simulink model "Satellite_Attitude_Model"  (R2018b)
settings: Solver=ode23tb  StartTime=0.0  StopTime=1000  FixedStep=0.001  RelTol=1e-4
values from neighbouring files (symbols this model uses):
  A = [A11, A12; A21, A22]    [Satellite_Attitude_Model_Parameters.m]
  ArgOfPerigee_init = deg2rad (TLE_degree(5))    [Satellite_Attitude_Model_Parameters.m]
  b = 10e-6    (= 1e-05)    [Satellite_Attitude_Model_Parameters.m]
  B = [B11,B12; B21,B22]    [Satellite_Attitude_Model_Parameters.m]
  D = 0    [Satellite_Attitude_Model_Parameters.m]
  eccentricity_init = TLE_degree(4)    [Satellite_Attitude_Model_Parameters.m]
  Hconf4 = [Hgyro;Hstr]    [Satellite_Attitude_Model_Parameters.m]
  inclination_init = deg2rad (TLE_degree(2))    [Satellite_Attitude_Model_Parameters.m]
  Km = 0.1    [Satellite_Attitude_Model_Parameters.m]
  Kt = 0.1    [Satellite_Attitude_Model_Parameters.m]
  L = 5.2e-3    (= 0.0052)    [Satellite_Attitude_Model_Parameters.m]
  MeanAnomaly_init = deg2rad (TLE_degree(6))    [Satellite_Attitude_Model_Parameters.m]
  meanMotion_init = meanMotion_init*2*pi/86400    [Satellite_Attitude_Model_Parameters.m]
  Q = 1e-10    [Satellite_Attitude_Model_Parameters.m]
  q_init = [0; 0; 0; 1]    [Satellite_Attitude_Model_Parameters.m]
  R = 2    [Satellite_Attitude_Model_Parameters.m]    (also in dynamicFunctions2.m = 7078000)
  RAAN_init = deg2rad (TLE_degree(3))    [Satellite_Attitude_Model_Parameters.m]
  Rconf4 = [diag(ones(3,1))*Rgyro zeros(3,4);         zeros(4,3) diag(ones(1,4))*Rstr]    [Satellite_Attitude_Model_Parameters.m]
  Rgyro = 1e-12    [Satellite_Attitude_Model_Parameters.m]
  Rstr = 1e-12    [Satellite_Attitude_Model_Parameters.m]
  rw_Inertia = 5e-4    (= 0.0005)    [Satellite_Attitude_Model_Parameters.m]
  RW_Mmax = 0.015    [Satellite_Attitude_Model_Parameters.m]
  rw_SensorToBody = [0 0.4741 0.4741 -0.9482;                   -0.9999 0.3333 0.3333 0.3333;                    0 -0.8165 0.8165 0 ]    [Satellite_Attitude_Model_Parameters.m]
  RW_wmax = 300    [Satellite_Attitude_Model_Parameters.m]
  satInertia = [Isx 0 0 ; 0 Isy 0 ; 0 0 Isz]    [Satellite_Attitude_Model_Parameters.m]    (also in dynamicFunctions2.m = diag([Isx Isy Isz]))
  semimajor_init = sqrt(mu_earth^(1/3)/meanMotion_init^(2/3))    [Satellite_Attitude_Model_Parameters.m]
  Ts = 0.01    [Satellite_Attitude_Model_Parameters.m]
  unit7 = ones(7,1)    [Satellite_Attitude_Model_Parameters.m]
  w_dot_init = [0;0;0]    [Satellite_Attitude_Model_Parameters.m]
  w_init = [0; 0; 0]    [Satellite_Attitude_Model_Parameters.m]
  wRW_init = [0;0;0;0]    [Satellite_Attitude_Model_Parameters.m]
undefined symbols (not defined in the file or in its folder): Continuous, Earth, Time, WGS84
libraries: simulink x14, simulink_extras x13, sharedtransform x8, aerolibutil x2, sharedTrackingLibrary x1, ctrlSharedLib x1, aerolibtransform2 x1, aerolibgravity2 x1
(part 2 of 3)

== system Satellite_Attitude_Model/Actuator Model (RW)/RW1 - DC Motor Controller3 ==
  RW1_Hdot_des : Inport
  Gain1 : Gain  Gain=12
  Gain2 : Gain  Gain=1/rw_Inertia
  Integrator : Integrator
  Mux : Mux  Inputs=2
  RW - DC Motor Model : Subsystem
  "Scope Desired and controlled RW-angular speed " : Scope
  Speed Controller1 : simulink/Continuous/PID Controller  Controller=PID  Form=Parallel  TimeDomain=Continuous-time  SampleTime=0.01  IntegratorMethod=Forward Euler  FilterMethod=Forward Euler  ControllerParametersSource=internal  P=9.56052273582853  I=13.4366327144231  D=1.16248121318414  UseFilter=on  N=2668.95305381072  TunerSelectOption=Transfer Function Based (PID Tuner App)  InitialConditionSource=internal  InitialConditionForIntegrator=0  InitialConditionForFilter=0  DifferentiatorICPrevScaledInput=0  ExternalReset=none  TrackingMode=off  Kt=1  LimitOutput=off  UpperSaturationLimit=inf  LowerSaturationLimit=-inf  LinearizeAsGain=on  AntiWindupMode=none  Kb=1  POutMin=[]  POutMax=[]  IOutMin=[]  IOutMax=[]  DOutMin=[]  DOutMax=[]  NOutMin=[]  NOutMax=[]  SumOutMin=[]  SumOutMax=[]  SaturationOutMin=[]  SaturationOutMax=[]  PParamMin=[]  PParamMax=[]  IParamMin=[]  IParamMax=[]  DParamMin=[]  DParamMax=[]  NParamMin=[]  NParamMax=[]  KbParamMin=[]  KbParamMax=[]  KtParamMin=[]  KtParamMax=[]  KbOutMin=[]  KbOutMax=[]  KtOutMin=[]  KtOutMax=[]  IntegratorOutMin=[]  IntegratorOutMax=[]  FilterOutMin=[]  FilterOutMax=[]  SumI1OutMin=[]  SumI1OutMax=[]  SumI2OutMin=[]  SumI2OutMax=[]  SumI3OutMin=[]  SumI3OutMax=[]  SumI4OutMin=[]  SumI4OutMax=[]  SumDOutMin=[]  SumDOutMax=[]  DifferentiatorOutMin=[]  DifferentiatorOutMax=[]  FilterDiffOutCoefMin=[]  FilterDiffOutCoefMax=[]  ReciprocalOutMin=[]  ReciprocalOutMax=[]  SumDenOutMin=[]  SumDenOutMax=[]  SumNumOutMin=[]  SumNumOutMax=[]  DivideOutMin=[]  DivideOutMax=[]  IntegratorContinuousStateAttributes=''  IntegratorStateMustResolveToSignalObject=off  IntegratorRTWStateStorageClass=Auto  FilterContinuousStateAttributes=''  FilterStateMustResolveToSignalObject=off  FilterRTWStateStorageClass=Auto  ParallelPVariant=InternalParameters  IdealPVariant=Disabled  IVariant=InternalParameters  DVariant=InternalParameters  IntegratorVariant=Continuous  SatVariant=Disabled  AWVariant=Passthrough  PCopyVariant=Disabled  TRVariant=Disabled  FdbkBlocksVariant=Forward  IdealPFdbkVariant=Disabled  SatFdbkVariant=Disabled  DerivativeFilterVariant=ContFilter  NVariant=InternalParameters  NCopyVariant=Disabled  FilterICVariant=InternalICsFilter  IntegratorICVariant=InternalICs  ExternalResetVariant=Disabled  TRSumVariant=Passthrough  SumFdbkVariant=Disabled  SumVariant=Sum_PID
  Sum1 : Sum  Inputs=|+-
  Sum2 : Sum  Inputs=|+-
  Torque Controller : simulink/Continuous/PID Controller  Controller=PID  Form=Parallel  TimeDomain=Continuous-time  SampleTime=0.01  IntegratorMethod=Forward Euler  FilterMethod=Forward Euler  ControllerParametersSource=internal  P=2.50374683332827e-05  I=0.022215359014968  D=0  UseFilter=on  N=100  TunerSelectOption=Transfer Function Based (PID Tuner App)  InitialConditionSource=internal  InitialConditionForIntegrator=0  InitialConditionForFilter=0  DifferentiatorICPrevScaledInput=0  ExternalReset=none  TrackingMode=off  Kt=1  LimitOutput=off  UpperSaturationLimit=inf  LowerSaturationLimit=-inf  LinearizeAsGain=on  AntiWindupMode=none  Kb=1  POutMin=[]  POutMax=[]  IOutMin=[]  IOutMax=[]  DOutMin=[]  DOutMax=[]  NOutMin=[]  NOutMax=[]  SumOutMin=[]  SumOutMax=[]  SaturationOutMin=[]  SaturationOutMax=[]  PParamMin=[]  PParamMax=[]  IParamMin=[]  IParamMax=[]  DParamMin=[]  DParamMax=[]  NParamMin=[]  NParamMax=[]  KbParamMin=[]  KbParamMax=[]  KtParamMin=[]  KtParamMax=[]  KbOutMin=[]  KbOutMax=[]  KtOutMin=[]  KtOutMax=[]  IntegratorOutMin=[]  IntegratorOutMax=[]  FilterOutMin=[]  FilterOutMax=[]  SumI1OutMin=[]  SumI1OutMax=[]  SumI2OutMin=[]  SumI2OutMax=[]  SumI3OutMin=[]  SumI3OutMax=[]  SumI4OutMin=[]  SumI4OutMax=[]  SumDOutMin=[]  SumDOutMax=[]  DifferentiatorOutMin=[]  DifferentiatorOutMax=[]  FilterDiffOutCoefMin=[]  FilterDiffOutCoefMax=[]  ReciprocalOutMin=[]  ReciprocalOutMax=[]  SumDenOutMin=[]  SumDenOutMax=[]  SumNumOutMin=[]  SumNumOutMax=[]  DivideOutMin=[]  DivideOutMax=[]  IntegratorContinuousStateAttributes=''  IntegratorStateMustResolveToSignalObject=off  IntegratorRTWStateStorageClass=Auto  FilterContinuousStateAttributes=''  FilterStateMustResolveToSignalObject=off  FilterRTWStateStorageClass=Auto  ParallelPVariant=InternalParameters  IdealPVariant=Disabled  IVariant=InternalParameters  DVariant=InternalParameters  IntegratorVariant=Continuous  SatVariant=Disabled  AWVariant=Passthrough  PCopyVariant=Disabled  TRVariant=Disabled  FdbkBlocksVariant=Forward  IdealPFdbkVariant=Disabled  SatFdbkVariant=Disabled  DerivativeFilterVariant=ContFilter  NVariant=InternalParameters  NCopyVariant=Disabled  FilterICVariant=InternalICsFilter  IntegratorICVariant=InternalICs  ExternalResetVariant=Disabled  TRSumVariant=Passthrough  SumFdbkVariant=Disabled  SumVariant=Sum_PID
  V limit : Saturate  UpperLimit=20  LowerLimit=-20
  w limit : Saturate  UpperLimit=RW_wmax  LowerLimit=-RW_wmax
  RW1_H : Outport
  RW1_w : Outport  Port=2
  RW1_Hdot : Outport  Port=3
  wires:
  Torque Controller/1 -> V limit/1
  RW - DC Motor Model/3(RW_Hrw_dot) -> RW1_Hdot/1, Sum1/2
  Mux/1 -> "Scope Desired and controlled RW-angular speed "/1
  V limit/1 -> Gain1/1
  Gain1/1 -> RW - DC Motor Model/1(V-rw)  "V-rw"
  RW - DC Motor Model/2(RW_w) -> RW1_w/1, Sum2/2, Mux/2
  Sum1/1 -> Torque Controller/1
  RW - DC Motor Model/1(RW_Hrw) -> RW1_H/1
  Speed Controller1/1 -> w limit/1
  w limit/1 -> Sum1/1
  Sum2/1 -> Speed Controller1/1  "M-error"
  Integrator/1 -> Gain2/1
  RW1_Hdot_des/1 -> Integrator/1
  Gain2/1 -> Mux/1, Sum2/1

== system Satellite_Attitude_Model/Actuator Model (RW)/RW1 - DC Motor Controller5 ==
  RW1_Hdot_des : Inport
  Gain1 : Gain  Gain=12
  Gain2 : Gain  Gain=1/rw_Inertia
  Integrator : Integrator
  Mux : Mux  Inputs=2
  RW - DC Motor Model : Subsystem
  "Scope Desired and controlled RW-angular speed " : Scope
  Speed Controller1 : simulink/Continuous/PID Controller  Controller=PID  Form=Parallel  TimeDomain=Continuous-time  SampleTime=0.01  IntegratorMethod=Forward Euler  FilterMethod=Forward Euler  ControllerParametersSource=internal  P=9.56052273582853  I=13.4366327144231  D=1.16248121318414  UseFilter=on  N=2668.95305381072  TunerSelectOption=Transfer Function Based (PID Tuner App)  InitialConditionSource=internal  InitialConditionForIntegrator=0  InitialConditionForFilter=0  DifferentiatorICPrevScaledInput=0  ExternalReset=none  TrackingMode=off  Kt=1  LimitOutput=off  UpperSaturationLimit=inf  LowerSaturationLimit=-inf  LinearizeAsGain=on  AntiWindupMode=none  Kb=1  POutMin=[]  POutMax=[]  IOutMin=[]  IOutMax=[]  DOutMin=[]  DOutMax=[]  NOutMin=[]  NOutMax=[]  SumOutMin=[]  SumOutMax=[]  SaturationOutMin=[]  SaturationOutMax=[]  PParamMin=[]  PParamMax=[]  IParamMin=[]  IParamMax=[]  DParamMin=[]  DParamMax=[]  NParamMin=[]  NParamMax=[]  KbParamMin=[]  KbParamMax=[]  KtParamMin=[]  KtParamMax=[]  KbOutMin=[]  KbOutMax=[]  KtOutMin=[]  KtOutMax=[]  IntegratorOutMin=[]  IntegratorOutMax=[]  FilterOutMin=[]  FilterOutMax=[]  SumI1OutMin=[]  SumI1OutMax=[]  SumI2OutMin=[]  SumI2OutMax=[]  SumI3OutMin=[]  SumI3OutMax=[]  SumI4OutMin=[]  SumI4OutMax=[]  SumDOutMin=[]  SumDOutMax=[]  DifferentiatorOutMin=[]  DifferentiatorOutMax=[]  FilterDiffOutCoefMin=[]  FilterDiffOutCoefMax=[]  ReciprocalOutMin=[]  ReciprocalOutMax=[]  SumDenOutMin=[]  SumDenOutMax=[]  SumNumOutMin=[]  SumNumOutMax=[]  DivideOutMin=[]  DivideOutMax=[]  IntegratorContinuousStateAttributes=''  IntegratorStateMustResolveToSignalObject=off  IntegratorRTWStateStorageClass=Auto  FilterContinuousStateAttributes=''  FilterStateMustResolveToSignalObject=off  FilterRTWStateStorageClass=Auto  ParallelPVariant=InternalParameters  IdealPVariant=Disabled  IVariant=InternalParameters  DVariant=InternalParameters  IntegratorVariant=Continuous  SatVariant=Disabled  AWVariant=Passthrough  PCopyVariant=Disabled  TRVariant=Disabled  FdbkBlocksVariant=Forward  IdealPFdbkVariant=Disabled  SatFdbkVariant=Disabled  DerivativeFilterVariant=ContFilter  NVariant=InternalParameters  NCopyVariant=Disabled  FilterICVariant=InternalICsFilter  IntegratorICVariant=InternalICs  ExternalResetVariant=Disabled  TRSumVariant=Passthrough  SumFdbkVariant=Disabled  SumVariant=Sum_PID
  Sum1 : Sum  Inputs=|+-
  Sum2 : Sum  Inputs=|+-
  Torque Controller : simulink/Continuous/PID Controller  Controller=PID  Form=Parallel  TimeDomain=Continuous-time  SampleTime=0.01  IntegratorMethod=Forward Euler  FilterMethod=Forward Euler  ControllerParametersSource=internal  P=2.50374683332827e-05  I=0.022215359014968  D=0  UseFilter=on  N=100  TunerSelectOption=Transfer Function Based (PID Tuner App)  InitialConditionSource=internal  InitialConditionForIntegrator=0  InitialConditionForFilter=0  DifferentiatorICPrevScaledInput=0  ExternalReset=none  TrackingMode=off  Kt=1  LimitOutput=off  UpperSaturationLimit=inf  LowerSaturationLimit=-inf  LinearizeAsGain=on  AntiWindupMode=none  Kb=1  POutMin=[]  POutMax=[]  IOutMin=[]  IOutMax=[]  DOutMin=[]  DOutMax=[]  NOutMin=[]  NOutMax=[]  SumOutMin=[]  SumOutMax=[]  SaturationOutMin=[]  SaturationOutMax=[]  PParamMin=[]  PParamMax=[]  IParamMin=[]  IParamMax=[]  DParamMin=[]  DParamMax=[]  NParamMin=[]  NParamMax=[]  KbParamMin=[]  KbParamMax=[]  KtParamMin=[]  KtParamMax=[]  KbOutMin=[]  KbOutMax=[]  KtOutMin=[]  KtOutMax=[]  IntegratorOutMin=[]  IntegratorOutMax=[]  FilterOutMin=[]  FilterOutMax=[]  SumI1OutMin=[]  SumI1OutMax=[]  SumI2OutMin=[]  SumI2OutMax=[]  SumI3OutMin=[]  SumI3OutMax=[]  SumI4OutMin=[]  SumI4OutMax=[]  SumDOutMin=[]  SumDOutMax=[]  DifferentiatorOutMin=[]  DifferentiatorOutMax=[]  FilterDiffOutCoefMin=[]  FilterDiffOutCoefMax=[]  ReciprocalOutMin=[]  ReciprocalOutMax=[]  SumDenOutMin=[]  SumDenOutMax=[]  SumNumOutMin=[]  SumNumOutMax=[]  DivideOutMin=[]  DivideOutMax=[]  IntegratorContinuousStateAttributes=''  IntegratorStateMustResolveToSignalObject=off  IntegratorRTWStateStorageClass=Auto  FilterContinuousStateAttributes=''  FilterStateMustResolveToSignalObject=off  FilterRTWStateStorageClass=Auto  ParallelPVariant=InternalParameters  IdealPVariant=Disabled  IVariant=InternalParameters  DVariant=InternalParameters  IntegratorVariant=Continuous  SatVariant=Disabled  AWVariant=Passthrough  PCopyVariant=Disabled  TRVariant=Disabled  FdbkBlocksVariant=Forward  IdealPFdbkVariant=Disabled  SatFdbkVariant=Disabled  DerivativeFilterVariant=ContFilter  NVariant=InternalParameters  NCopyVariant=Disabled  FilterICVariant=InternalICsFilter  IntegratorICVariant=InternalICs  ExternalResetVariant=Disabled  TRSumVariant=Passthrough  SumFdbkVariant=Disabled  SumVariant=Sum_PID
  V limit : Saturate  UpperLimit=20  LowerLimit=-20
  w limit : Saturate  UpperLimit=RW_wmax  LowerLimit=-RW_wmax
  RW1_H : Outport
  RW1_w : Outport  Port=2
  RW1_Hdot : Outport  Port=3
  wires:
  Torque Controller/1 -> V limit/1
  RW - DC Motor Model/3(RW_Hrw_dot) -> RW1_Hdot/1, Sum1/2
  Mux/1 -> "Scope Desired and controlled RW-angular speed "/1
  V limit/1 -> Gain1/1
  Gain1/1 -> RW - DC Motor Model/1(V-rw)  "V-rw"
  RW - DC Motor Model/2(RW_w) -> RW1_w/1, Sum2/2, Mux/2
  Sum1/1 -> Torque Controller/1
  RW - DC Motor Model/1(RW_Hrw) -> RW1_H/1
  Speed Controller1/1 -> w limit/1
  w limit/1 -> Sum1/1
  Sum2/1 -> Speed Controller1/1  "M-error"
  Integrator/1 -> Gain2/1
  RW1_Hdot_des/1 -> Integrator/1
  Gain2/1 -> Mux/1, Sum2/1

== system Satellite_Attitude_Model/Julian Date Model/Time To Julian Date Model ==
  time : Inport
  Date To Julian Date Model : MATLAB Function  TreatAsAtomicUnit=on
  JulianDate : Outport
  wires:
  time/1 -> Date To Julian Date Model/1(time)
  Date To Julian Date Model/1(JD) -> JulianDate/1

== system Satellite_Attitude_Model/Orbit Propagator Model/Mean Motion To Semi-major Axis ==
  In1 : Inport
  MATLAB Function : MATLAB Function  TreatAsAtomicUnit=on
  Out1 : Outport
  wires:
  In1/1 -> MATLAB Function/1(a)
  MATLAB Function/1(meanMotion) -> Out1/1

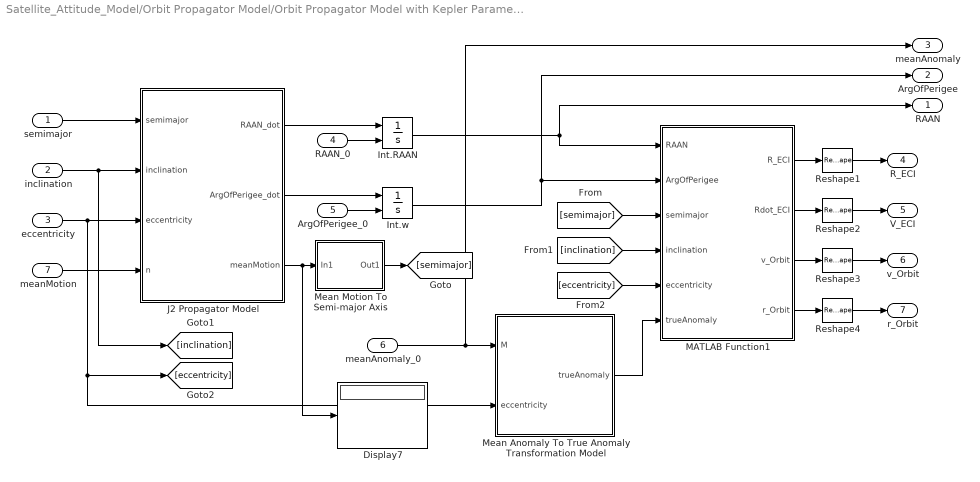
== system Satellite_Attitude_Model/Orbit Propagator Model/Orbit Propagator Model with Kepler Parameters(ECI) ==
  semimajor : Inport
  inclination : Inport  Port=2
  eccentricity : Inport  Port=3
  RAAN_0 : Inport  Port=4
  ArgOfPerigee_0 : Inport  Port=5
  meanAnomaly_0 : Inport  Port=6
  meanMotion : Inport  Port=7
  Display7 : Display
  Int.RAAN : Integrator  InitialConditionSource=external
  Int.w : Integrator  InitialConditionSource=external
  J2 Propagator Model : MATLAB Function  TreatAsAtomicUnit=on
  MATLAB Function1 : MATLAB Function  TreatAsAtomicUnit=on
  Mean Anomaly To True Anomaly Transformation Model : MATLAB Function  TreatAsAtomicUnit=on
  Mean Motion To Semi-major Axis : Subsystem
  Reshape{1..4} (4 alike) : Reshape  OutputDimensionality=Column vector (2-D)
  RAAN : Outport
  ArgOfPerigee : Outport  Port=2
  meanAnomaly : Outport  Port=3
  R_ECI : Outport  Port=4
  V_ECI : Outport  Port=5
  v_Orbit : Outport  Port=6
  r_Orbit : Outport  Port=7
  wires:
  ArgOfPerigee_0/1 -> Int.w/2
  RAAN_0/1 -> Int.RAAN/2
  semimajor/1 -> J2 Propagator Model/1(semimajor)
  J2 Propagator Model/2(ArgOfPerigee_dot) -> Int.w/1
  J2 Propagator Model/1(RAAN_dot) -> Int.RAAN/1
  Int.RAAN/1 -> MATLAB Function1/1(RAAN), RAAN/1
  Int.w/1 -> ArgOfPerigee/1, MATLAB Function1/2(ArgOfPerigee)
  meanAnomaly_0/1 -> meanAnomaly/1, Mean Anomaly To True Anomaly Transformation Model/1(M)
  inclination/1 -> [inclination], J2 Propagator Model/2(inclination)
  eccentricity/1 -> Mean Anomaly To True Anomaly Transformation Model/2(eccentricity), [eccentricity], J2 Propagator Model/3(eccentricity)
  Mean Anomaly To True Anomaly Transformation Model/1(trueAnomaly) -> MATLAB Function1/6(trueAnomaly)
  MATLAB Function1/2(Rdot_ECI) -> Reshape2/1
  MATLAB Function1/1(R_ECI) -> Reshape1/1
  Reshape2/1 -> V_ECI/1
  Reshape1/1 -> R_ECI/1
  [semimajor] -> MATLAB Function1/3(semimajor)
  [inclination] -> MATLAB Function1/4(inclination)
  [eccentricity] -> MATLAB Function1/5(eccentricity)
  MATLAB Function1/3(v_Orbit) -> Reshape3/1
  Reshape3/1 -> v_Orbit/1
  MATLAB Function1/4(r_Orbit) -> Reshape4/1
  Reshape4/1 -> r_Orbit/1
  meanMotion/1 -> J2 Propagator Model/4(n)
  Mean Motion To Semi-major Axis/1(Out1) -> [semimajor]
  J2 Propagator Model/3(meanMotion) -> Display7/1, Mean Motion To Semi-major Axis/1(In1)

== system Satellite_Attitude_Model/Orbit Propagator Model/True Anomaly to Mean Anomaly ==
  ecc : Inport
  TrAn : Inport  Port=2
  True Anomaly to Mean Anomaly : MATLAB Function  TreatAsAtomicUnit=on
  Out1 : Outport
  wires:
  TrAn/1 -> True Anomaly to Mean Anomaly/2(TrAn)
  ecc/1 -> True Anomaly to Mean Anomaly/1(ecc)
  True Anomaly to Mean Anomaly/1(M) -> Out1/1

== system Satellite_Attitude_Model/Satellite Kinematic & Dynamic Model/Dynamic Model ==
  Mc+Md : Inport
  "Hrw_B " : Inport  Port=2
  Add : Sum  Inputs=-+
  Add1 : Sum
  Embedded MATLAB Function : MATLAB Function  TreatAsAtomicUnit=on
  IC : InitialCondition  Value=w_init
  IC1 : InitialCondition  Value=w_dot_init
  Inertia Matrix : Constant  Value=satInertia  VectorParams1D=off
  Integrator : Integrator  InitialConditionSource=external  InitialCondition=[0;0;0]
  Invert 3x3 Matrix : aerolibutil/Invert  3x3 Matrix
  Product : Product  Multiplication=Matrix(*)  RndMeth=Zero
  Product1 : Product  Multiplication=Matrix(*)  RndMeth=Zero
  Reshape : Reshape  OutputDimensionality=Column vector (2-D)
  Reshape1 : Reshape  OutputDimensionality=Column vector (2-D)
  w_initial : Constant  Value=w_init  VectorParams1D=off  SampleTime=-1
  w_IB_B : Outport
  wires:
  Inertia Matrix/1 -> Invert 3x3 Matrix/1, Product/1
  IC/1 -> Product/2, Embedded MATLAB Function/1(w)
  Mc+Md/1 -> Reshape1/1
  Invert 3x3 Matrix/1 -> Product1/1
  Integrator/1 -> w_IB_B/1, IC/1
  Product1/1 -> IC1/1
  Embedded MATLAB Function/1(y) -> Reshape/1
  w_initial/1 -> Integrator/2
  Add/1 -> Product1/2
  IC1/1 -> Integrator/1
  Reshape/1 -> Add/1
  Reshape1/1 -> Add/2
  Product/1 -> Add1/1
  Add1/1 -> Embedded MATLAB Function/2(Iw_plus_hwheel)
  "Hrw_B "/1 -> Add1/2

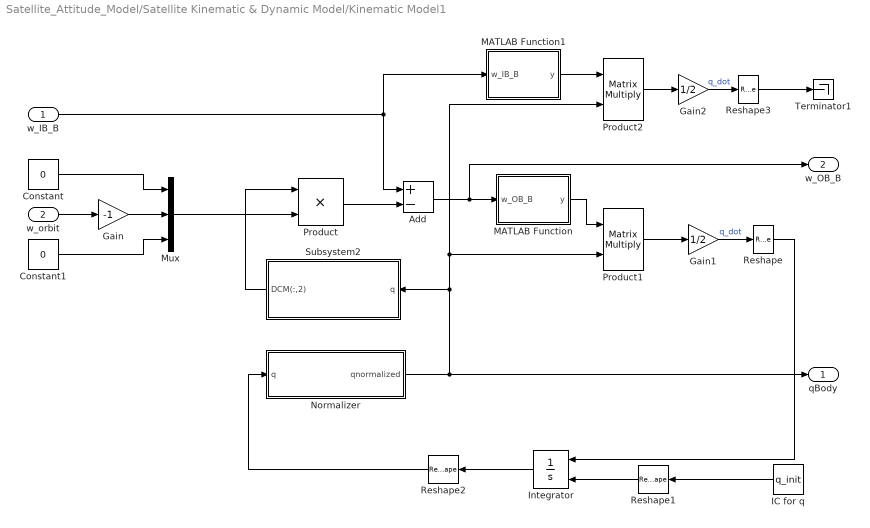
== system Satellite_Attitude_Model/Satellite Kinematic & Dynamic Model/Kinematic Model1 ==
  w_IB_B : Inport
  w_orbit : Inport  Port=2
  Add : Sum  Inputs=+-
  Constant : Constant  Value=0
  Constant1 : Constant  Value=0
  Gain : Gain  Gain=-1
  Gain1 : Gain  Gain=1/2
  Gain2 : Gain  Gain=1/2
  IC for q : Constant  Value=q_init  SampleTime=Ts
  Integrator : Integrator  InitialConditionSource=external
  MATLAB Function : MATLAB Function  TreatAsAtomicUnit=on
  MATLAB Function1 : MATLAB Function  TreatAsAtomicUnit=on
  Mux : Mux  Inputs=3
  Normalizer : MATLAB Function  TreatAsAtomicUnit=on
  Product : Product
  Product1 : Product  Multiplication=Matrix(*)
  Product2 : Product  Multiplication=Matrix(*)
  Reshape{,1..3} (4 alike) : Reshape  OutputDimensionality=Column vector (2-D)
  Subsystem2 : Subsystem
  Terminator1 : Terminator
  qBody : Outport
  w_OB_B : Outport  Port=2
  wires:
  Reshape2/1 -> Normalizer/1(q)
  Product/1 -> Add/2
  Integrator/1 -> Reshape2/1
  Normalizer/1(qnormalized) -> qBody/1, Subsystem2/1(q), Product1/2, Product2/2
  IC for q/1 -> Reshape1/1
  Reshape1/1 -> Integrator/2
  Add/1 -> MATLAB Function/1(w_OB_B), w_OB_B/1
  w_orbit/1 -> Gain/1
  Mux/1 -> Product/2
  Constant/1 -> Mux/1
  Constant1/1 -> Mux/3
  Product1/1 -> Gain1/1
  MATLAB Function/1(y) -> Product1/1
  Gain1/1 -> Reshape/1  "q_dot"
  w_IB_B/1 -> MATLAB Function1/1(w_IB_B), Add/1
  Product2/1 -> Gain2/1
  MATLAB Function1/1(y) -> Product2/1
  Gain2/1 -> Reshape3/1  "q_dot"
  Subsystem2/1(DCM(:,2)) -> Product/1
  Gain/1 -> Mux/2
  Reshape/1 -> Integrator/1
  Reshape3/1 -> Terminator1/1

== system Satellite_Attitude_Model/Satellite Kinematic & Dynamic Model/Subsystem ==
  qest : Inport
  Quaternions to Direction Cosine Matrix : sharedtransform/Quaternions to  Direction Cosine Matrix  aMode=aMode
      settings: SourceProductName=Aerospace Blockset  SourceProductBaseCode=AE
  Subsystem : Subsystem
  "DCM " : Outport
  wires:
  Quaternions to Direction Cosine Matrix/1 -> "DCM "/1
  Subsystem/1(q0,q1,q2,q3) -> Quaternions to Direction Cosine Matrix/1
  qest/1 -> Subsystem/1(q1,q2,q3,q4)

== system Satellite_Attitude_Model/Satellite Kinematic & Dynamic Model/Subsystem1 ==
  "DCM " : Inport
  Direction Cosine Matrix to Rotation Angles : sharedtransform/Direction Cosine Matrix to Rotation Angles  rotationOrder=ZYX  aMode=aMode  action=None  tolerance=eps(2)
      settings: SourceProductName=Aerospace Blockset  SourceProductBaseCode=AE
  Radians to Degrees1 : simulink_extras/Transformations/Radians to Degrees
  Euler Angle : Outport
  wires:
  Radians to Degrees1/1 -> Euler Angle/1
  Direction Cosine Matrix to Rotation Angles/1 -> Radians to Degrees1/1
  "DCM "/1 -> Direction Cosine Matrix to Rotation Angles/1

== system Satellite_Attitude_Model/Sensor Measurement Model (GYRO + STR)/GYRO Sensor Model ==
  w_Body : Inport
  Gyroscope Model : Subsystem
  Zero-Order Hold2 : ZeroOrderHold  SampleTime=Ts
  w_Body_meas : Outport
  wires:
  w_Body/1 -> Gyroscope Model/1(w_Body)
  Gyroscope Model/1(Gyro1_wmeas) -> Zero-Order Hold2/1
  Zero-Order Hold2/1 -> w_Body_meas/1

== system Satellite_Attitude_Model/Sensor Measurement Model (GYRO + STR)/Normalization Model ==
  u : Inport
  Divide : Product  Inputs=*/
  MATLAB Function : MATLAB Function  TreatAsAtomicUnit=on
  Math Function2 : Math  Operator=square  SaturateOnIntegerOverflow=on
  Sum of Elements : Sum  Inputs=+
  Normalized_u : Outport
  wires:
  Divide/1 -> Normalized_u/1
  MATLAB Function/1(y) -> Divide/2
  Sum of Elements/1 -> MATLAB Function/1(u)
  u/1 -> Divide/1, Math Function2/1
  Math Function2/1 -> Sum of Elements/1

== system Satellite_Attitude_Model/Sensor Measurement Model (GYRO + STR)/Star Tracker Model ==
  q_Body : Inport
  Scope : Scope
  StarTracker 1 Error Model3 : Subsystem  TreatAsAtomicUnit=on
  Zero-Order Hold2 : ZeroOrderHold  SampleTime=0.1
  q_Body_meas : Outport
  wires:
  Zero-Order Hold2/1 -> Scope/1, q_Body_meas/1
  q_Body/1 -> StarTracker 1 Error Model3/1("q_Body ")
  StarTracker 1 Error Model3/1("q_body_meas ") -> Zero-Order Hold2/1

== system Satellite_Attitude_Model/Subsystem/Subsystem1 ==
  q0,q1,q2,q3 : Inport
  Demux1 : Demux
  Mux1 : Mux
  q1,q2,q3,q4 : Outport
  wires:
  q0,q1,q2,q3/1 -> Demux1/1
  Mux1/1 -> q1,q2,q3,q4/1
  Demux1/1 -> Mux1/4
  Demux1/2 -> Mux1/1
  Demux1/3 -> Mux1/2
  Demux1/4 -> Mux1/3

== system Satellite_Attitude_Model/Subsystem2/Subsystem ==
  qest : Inport
  Demux2 : Demux
  Mux2 : Mux
  Quaternions to Direction Cosine Matrix : sharedtransform/Quaternions to  Direction Cosine Matrix  aMode=aMode
      settings: SourceProductName=Aerospace Blockset  SourceProductBaseCode=AE
  "DCM " : Outport
  wires:
  Mux2/1 -> Quaternions to Direction Cosine Matrix/1
  Quaternions to Direction Cosine Matrix/1 -> "DCM "/1
  Demux2/2 -> Mux2/3
  Demux2/4 -> Mux2/1
  Demux2/3 -> Mux2/4
  Demux2/1 -> Mux2/2
  qest/1 -> Demux2/1

== system Satellite_Attitude_Model/Sun Position Model/Subsystem1 ==
  JD2000 : Inport
  r_ECI : Inport  Port=2
  DCM_qECI : Inport  Port=3
  DCM_qBody : Inport  Port=4
  Display3 : Display
  Invert 3x3 Matrix : aerolibutil/Invert  3x3 Matrix
  Product : Product  Multiplication=Matrix(*)
  Product1 : Product  Multiplication=Matrix(*)
  "Sun Vector Model " : Subsystem
  SunVector_Orbit : Outport
  "sunVector_ECI " : Outport  Port=2
  wires:
  "Sun Vector Model "/1(sunVector_ECI) -> "sunVector_ECI "/1, Product/2, Display3/1
  JD2000/1 -> "Sun Vector Model "/1(JD2000)
  Product/1 -> Product1/2
  Product1/1 -> SunVector_Orbit/1
  Invert 3x3 Matrix/1 -> Product1/1
  DCM_qECI/1 -> Product/1
  DCM_qBody/1 -> Invert 3x3 Matrix/1
  r_ECI/1 -> "Sun Vector Model "/2(rECI)

== system Satellite_Attitude_Model/Total Disturbance Torque Model/Aerodynamic Disturbance Torque Model ==
  SC_Velocity_Orbit : Inport
  DCM : Inport  Port=2
  Aerodynamic Disturbance Torque Model : Subsystem
  Product : Product  Multiplication=Matrix(*)
  AerodynamicDistTorque_Orbit : Outport
  AerodynamicDistTorque_Body : Outport  Port=2
  wires:
  Aerodynamic Disturbance Torque Model/1(AerodynamicDistTorque) -> Product/2, AerodynamicDistTorque_Orbit/1
  Product/1 -> AerodynamicDistTorque_Body/1
  DCM/1 -> Product/1
  SC_Velocity_Orbit/1 -> Aerodynamic Disturbance Torque Model/1(SC_Velocity_Orbit)

== system Satellite_Attitude_Model/Total Disturbance Torque Model/Gravity Gradient Disturbance Torque Model ==
  w0 : Inport
  DCM : Inport  Port=2
  SatInertiaMatrix : Inport  Port=3
  Gain : Gain  Gain=3
  "Last Column " : MATLAB Function  TreatAsAtomicUnit=on
  Product : Product
  Product1 : Product
  Product2 : Product  Multiplication=Matrix(*)
  Product3 : Product  Multiplication=Matrix(*)
  Product4 : Product  Multiplication=Matrix(*)
  Skew Symmetric Matrix : MATLAB Function  TreatAsAtomicUnit=on
  GGDistTorque : Outport
  GGDistTorque_Body : Outport  Port=2
  wires:
  Gain/1 -> Product1/1
  Product2/1 -> Product3/2  "3x1"
  w0/1 -> Product/1, Product/2
  Product3/1 -> Product1/2
  Product1/1 -> Product4/2, GGDistTorque/1
  "Last Column "/1(LastColumn_DCM) -> Product2/2, Skew Symmetric Matrix/1(LastColumn_DCM)  "3x1"
  Product/1 -> Gain/1
  SatInertiaMatrix/1 -> Product2/1
  Skew Symmetric Matrix/1(SkewSym_DCM) -> Product3/1  "3x3"
  DCM/1 -> Product4/1, "Last Column "/1(DCM)
  Product4/1 -> GGDistTorque_Body/1

== system Satellite_Attitude_Model/Total Disturbance Torque Model/Magnetic Field Disturbance Torque Model ==
  LLA_degrees : Inport
  DCM_qBody : Inport  Port=2
  Subsystem : Subsystem
  MagFieldDistTorque_Orbit : Outport
  MagFieldDistTorque_Body : Outport  Port=2
  wires:
  Subsystem/1(MagField_Orbit) -> MagFieldDistTorque_Orbit/1
  Subsystem/2(MagField_Body) -> MagFieldDistTorque_Body/1
  LLA_degrees/1 -> Subsystem/1(LLA_degrees)
  DCM_qBody/1 -> Subsystem/2(DCM_qBody)

== system Satellite_Attitude_Model/Total Disturbance Torque Model/Solar Radiation Disturbance Torque Model ==
  SunVector_Orbit : Inport
  DCM : Inport  Port=2
  Product : Product  Multiplication=Matrix(*)
  Solar Radiation Disturbance Torque Model : Subsystem
  SolarRadDistTorque : Outport
  SolarRadDistTorque_Body : Outport  Port=2
  wires:
  SunVector_Orbit/1 -> Solar Radiation Disturbance Torque Model/1(SunPositionVector)
  Solar Radiation Disturbance Torque Model/1(SolarRadDistTorque) -> SolarRadDistTorque/1, Product/2
  Product/1 -> SolarRadDistTorque_Body/1
  DCM/1 -> Product/1

== system Satellite_Attitude_Model/Actuator Model (RW)/RW1 - DC Motor Controller1/RW - DC Motor Model ==
  V-rw : Inport
  Gain : Gain  Gain=Km
  Gain2 : Gain  Gain=Kt
  Gain6 : Gain  Gain=rw_Inertia
  M(s) --> w(s) : simulink_extras/Additional Linear/Transfer Fcn (with initial states)  N=[1]  D=[rw_Inertia b]  X0=0
  Sum3 : Sum  Inputs=|+-
  V(s) --> I(s) : simulink_extras/Additional Linear/Transfer Fcn (with initial states)  N=1  D=[L R]  X0=0
  w limit : Saturate  UpperLimit=RW_wmax  LowerLimit=-RW_wmax
  RW_Hrw : Outport
  RW_w : Outport  Port=2
  RW_Hrw_dot : Outport  Port=3
  wires:
  V-rw/1 -> Sum3/1
  Gain2/1 -> M(s) --> w(s)/1, RW_Hrw_dot/1  "M-rw"
  Gain6/1 -> RW_Hrw/1
  Gain/1 -> Sum3/2
  M(s) --> w(s)/1 -> w limit/1
  Sum3/1 -> V(s) --> I(s)/1  "V-rw"
  V(s) --> I(s)/1 -> Gain2/1
  w limit/1 -> RW_w/1, Gain6/1, Gain/1

== system Satellite_Attitude_Model/Actuator Model (RW)/RW1 - DC Motor Controller2/RW - DC Motor Model ==
  V-rw : Inport
  Gain : Gain  Gain=Km
  Gain2 : Gain  Gain=Kt
  Gain6 : Gain  Gain=rw_Inertia
  M(s) --> w(s) : simulink_extras/Additional Linear/Transfer Fcn (with initial states)  N=[1]  D=[rw_Inertia b]  X0=0
  Sum3 : Sum  Inputs=|+-
  V(s) --> I(s) : simulink_extras/Additional Linear/Transfer Fcn (with initial states)  N=1  D=[L R]  X0=0
  w limit : Saturate  UpperLimit=RW_wmax  LowerLimit=-RW_wmax
  RW_Hrw : Outport
  RW_w : Outport  Port=2
  RW_Hrw_dot : Outport  Port=3
  wires:
  V-rw/1 -> Sum3/1
  Gain2/1 -> M(s) --> w(s)/1, RW_Hrw_dot/1  "M-rw"
  Gain6/1 -> RW_Hrw/1
  Gain/1 -> Sum3/2
  M(s) --> w(s)/1 -> w limit/1
  Sum3/1 -> V(s) --> I(s)/1  "V-rw"
  V(s) --> I(s)/1 -> Gain2/1
  w limit/1 -> RW_w/1, Gain6/1, Gain/1

== system Satellite_Attitude_Model/Actuator Model (RW)/RW1 - DC Motor Controller3/RW - DC Motor Model ==
  V-rw : Inport
  Gain : Gain  Gain=Km
  Gain2 : Gain  Gain=Kt
  Gain6 : Gain  Gain=rw_Inertia
  M(s) --> w(s) : simulink_extras/Additional Linear/Transfer Fcn (with initial states)  N=[1]  D=[rw_Inertia b]  X0=0
  Sum3 : Sum  Inputs=|+-
  V(s) --> I(s) : simulink_extras/Additional Linear/Transfer Fcn (with initial states)  N=1  D=[L R]  X0=0
  w limit : Saturate  UpperLimit=RW_wmax  LowerLimit=-RW_wmax
  RW_Hrw : Outport
  RW_w : Outport  Port=2
  RW_Hrw_dot : Outport  Port=3
  wires:
  V-rw/1 -> Sum3/1
  Gain2/1 -> M(s) --> w(s)/1, RW_Hrw_dot/1  "M-rw"
  Gain6/1 -> RW_Hrw/1
  Gain/1 -> Sum3/2
  M(s) --> w(s)/1 -> w limit/1
  Sum3/1 -> V(s) --> I(s)/1  "V-rw"
  V(s) --> I(s)/1 -> Gain2/1
  w limit/1 -> RW_w/1, Gain6/1, Gain/1

== system Satellite_Attitude_Model/Actuator Model (RW)/RW1 - DC Motor Controller5/RW - DC Motor Model ==
  V-rw : Inport
  Gain : Gain  Gain=Km
  Gain2 : Gain  Gain=Kt
  Gain6 : Gain  Gain=rw_Inertia
  M(s) --> w(s) : simulink_extras/Additional Linear/Transfer Fcn (with initial states)  N=[1]  D=[rw_Inertia b]  X0=0
  Sum3 : Sum  Inputs=|+-
  V(s) --> I(s) : simulink_extras/Additional Linear/Transfer Fcn (with initial states)  N=1  D=[L R]  X0=0
  w limit : Saturate  UpperLimit=RW_wmax  LowerLimit=-RW_wmax
  RW_Hrw : Outport
  RW_w : Outport  Port=2
  RW_Hrw_dot : Outport  Port=3
  wires:
  V-rw/1 -> Sum3/1
  Gain2/1 -> M(s) --> w(s)/1, RW_Hrw_dot/1  "M-rw"
  Gain6/1 -> RW_Hrw/1
  Gain/1 -> Sum3/2
  M(s) --> w(s)/1 -> w limit/1
  Sum3/1 -> V(s) --> I(s)/1  "V-rw"
  V(s) --> I(s)/1 -> Gain2/1
  w limit/1 -> RW_w/1, Gain6/1, Gain/1

== system Satellite_Attitude_Model/Orbit Propagator Model/Orbit Propagator Model with Kepler Parameters(ECI)/Mean Motion To Semi-major Axis ==
  In1 : Inport
  MATLAB Function : MATLAB Function  TreatAsAtomicUnit=on
  Out1 : Outport
  wires:
  In1/1 -> MATLAB Function/1(n)
  MATLAB Function/1(semiMajor) -> Out1/1

== system Satellite_Attitude_Model/Satellite Kinematic & Dynamic Model/Kinematic Model1/Subsystem2 ==
  q : Inport
  MATLAB Function : MATLAB Function  TreatAsAtomicUnit=on
  Quaternions to Direction Cosine Matrix : sharedtransform/Quaternions to  Direction Cosine Matrix  aMode=aMode
      settings: SourceProductName=Aerospace Blockset  SourceProductBaseCode=AE
  Reshape2 : Reshape  OutputDimensionality=Column vector (2-D)
  Subsystem : Subsystem
  DCM(:,2) : Outport
  wires:
  Subsystem/1(q0,q1,q2,q3) -> Quaternions to Direction Cosine Matrix/1
  q/1 -> Subsystem/1(q1,q2,q3,q4)
  Quaternions to Direction Cosine Matrix/1 -> MATLAB Function/1(DCM)
  MATLAB Function/1(DCM_2) -> Reshape2/1
  Reshape2/1 -> DCM(:,2)/1

== system Satellite_Attitude_Model/Satellite Kinematic & Dynamic Model/Subsystem/Subsystem ==
  q1,q2,q3,q4 : Inport
  Demux1 : Demux
  Mux1 : Mux
  q0,q1,q2,q3 : Outport
  wires:
  Demux1/2 -> Mux1/3
  q1,q2,q3,q4/1 -> Demux1/1
  Mux1/1 -> q0,q1,q2,q3/1
  Demux1/4 -> Mux1/1
  Demux1/1 -> Mux1/2
  Demux1/3 -> Mux1/4

== system Satellite_Attitude_Model/Sensor Measurement Model (GYRO + STR)/GYRO Sensor Model/Gyroscope Model ==
  w_Body : Inport
  Add : Sum
  Band-Limited White Noise : simulink/Sources/Band-Limited White Noise  Cov=Rgyro*Ts  Ts=Ts  seed=[23341]
  Saturation1 : Saturate  UpperLimit=abs(1000)  LowerLimit=-abs(1000)
  Gyro1_wmeas : Outport
  wires:
  Add/1 -> Saturation1/1
  Saturation1/1 -> Gyro1_wmeas/1
  w_Body/1 -> Add/1
  Band-Limited White Noise/1 -> Add/2

== system Satellite_Attitude_Model/Sensor Measurement Model (GYRO + STR)/Star Tracker Model/StarTracker 1 Error Model3 ==
  "q_Body " : Inport
  Add : Sum
  Band-Limited White Noise : simulink/Sources/Band-Limited White Noise  Cov=Rstr*Ts  Ts=Ts  seed=[12345]
  "q_body_meas " : Outport
  wires:
  Band-Limited White Noise/1 -> Add/2
  "q_Body "/1 -> Add/1
  Add/1 -> "q_body_meas "/1

== system Satellite_Attitude_Model/Sun Position Model/Subsystem1/Sun Vector Model  ==
  JD2000 : Inport
  rECI : Inport  Port=2
  SunVectorModel : MATLAB Function  TreatAsAtomicUnit=on
  sunVector_ECI : Outport
  wires:
  rECI/1 -> SunVectorModel/2(rECI)
  SunVectorModel/1(sunVectorECI) -> sunVector_ECI/1
  JD2000/1 -> SunVectorModel/1(JD2000)

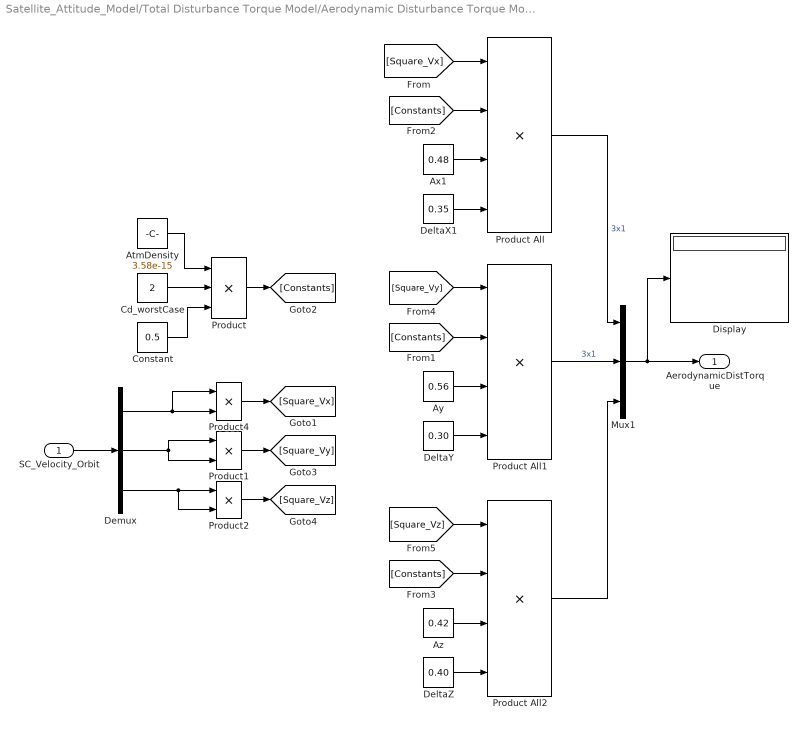
== system Satellite_Attitude_Model/Total Disturbance Torque Model/Aerodynamic Disturbance Torque Model/Aerodynamic Disturbance Torque Model ==
  SC_Velocity_Orbit : Inport
  AtmDensity : Constant  Value=3.58e-15
  Ax1 : Constant  Value=0.48
  Ay : Constant  Value=0.56
  Az : Constant  Value=0.42
  Cd_worstCase : Constant  Value=2
  Constant : Constant  Value=0.5
  DeltaX1 : Constant  Value=0.35
  DeltaY : Constant  Value=0.30
  DeltaZ : Constant  Value=0.40
  Demux : Demux  Outputs=3
  Display : Display
  Mux1 : Mux  Inputs=3
  Product : Product  Inputs=3
  Product All : Product  Inputs=4
  Product All1 : Product  Inputs=4
  Product All2 : Product  Inputs=4
  Product1 : Product
  Product2 : Product
  Product4 : Product
  AerodynamicDistTorque : Outport
  wires:
  Cd_worstCase/1 -> Product/2
  Constant/1 -> Product/3
  AtmDensity/1 -> Product/1
  [Square_Vx] -> Product All/1
  Ax1/1 -> Product All/3
  DeltaX1/1 -> Product All/4
  Product/1 -> [Constants]
  [Constants] -> Product All/2
  [Square_Vy] -> Product All1/1
  Ay/1 -> Product All1/3
  DeltaY/1 -> Product All1/4
  [Constants] -> Product All1/2
  [Square_Vz] -> Product All2/1
  Az/1 -> Product All2/3
  DeltaZ/1 -> Product All2/4
  [Constants] -> Product All2/2
  Product All/1 -> Mux1/1  "3x1"
  Product All1/1 -> Mux1/2  "3x1"
  Product All2/1 -> Mux1/3
  Mux1/1 -> AerodynamicDistTorque/1, Display/1
  SC_Velocity_Orbit/1 -> Demux/1
  Demux/1 -> Product4/1, Product4/2
  Demux/2 -> Product1/2, Product1/1
  Demux/3 -> Product2/2, Product2/1
  Product4/1 -> [Square_Vx]
  Product1/1 -> [Square_Vy]
  Product2/1 -> [Square_Vz]

== system Satellite_Attitude_Model/Total Disturbance Torque Model/Magnetic Field Disturbance Torque Model/Subsystem ==
  LLA_degrees : Inport
  DCM_qBody : Inport  Port=2
  Demux : Demux  Outputs=3
  Display3 : Display
  Gain2 : Gain  Gain=10^-9
  International Geomagnetic Reference Field 12 : aerolibgravity2/International Geomagnetic Reference Field 12  units=Metric (MKS)  time_in=off  month=January  day=1  year=2020  action=None  sv_out=off
      settings: SourceProductName=Aerospace Blockset  SourceProductBaseCode=AE
  Product4 : Product  Multiplication=Matrix(*)
  Terminator{2..5} (4 alike) : Terminator
  MagField_Orbit : Outport
  MagField_Body : Outport  Port=2
  wires:
  Demux/2 -> International Geomagnetic Reference Field 12/3
  Gain2/1 -> MagField_Orbit/1, Product4/2, Display3/1
  International Geomagnetic Reference Field 12/2 -> Terminator2/1
  International Geomagnetic Reference Field 12/1 -> Gain2/1
  Product4/1 -> MagField_Body/1
  International Geomagnetic Reference Field 12/4 -> Terminator4/1
  LLA_degrees/1 -> Demux/1
  Demux/3 -> International Geomagnetic Reference Field 12/1
  International Geomagnetic Reference Field 12/5 -> Terminator5/1
  International Geomagnetic Reference Field 12/3 -> Terminator3/1
  Demux/1 -> International Geomagnetic Reference Field 12/2
  DCM_qBody/1 -> Product4/1

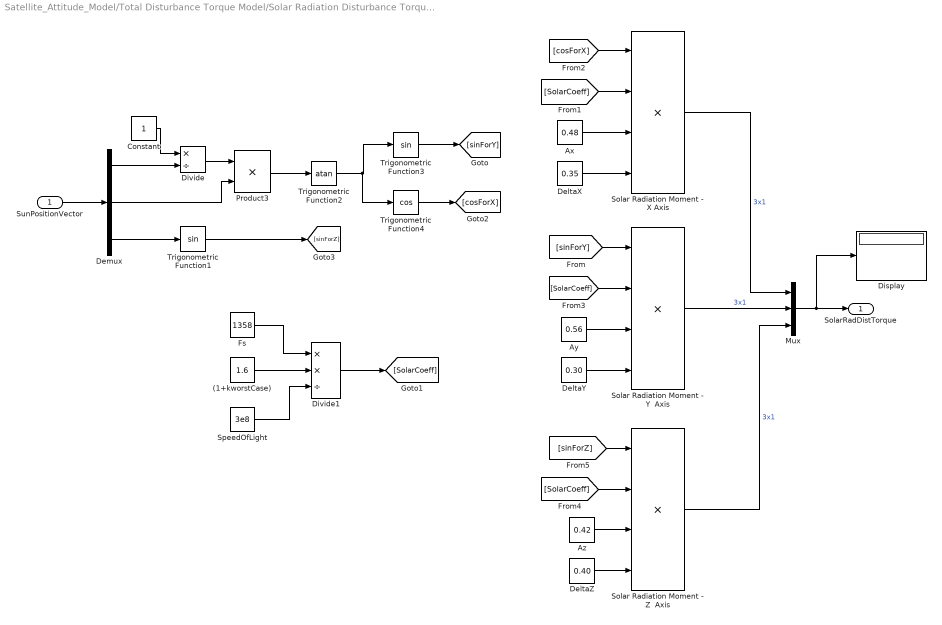
== system Satellite_Attitude_Model/Total Disturbance Torque Model/Solar Radiation Disturbance Torque Model/Solar Radiation Disturbance Torque Model ==
  SunPositionVector : Inport
  (1+kworstCase) : Constant  Value=1.6
  Ax : Constant  Value=0.48
  Ay : Constant  Value=0.56
  Az : Constant  Value=0.42
  Constant : Constant
  DeltaX : Constant  Value=0.35
  DeltaY : Constant  Value=0.30
  DeltaZ : Constant  Value=0.40
  Demux : Demux  Outputs=3
  Display : Display
  Divide : Product  Inputs=*/
  Divide1 : Product  Inputs=**/
  Fs : Constant  Value=1358
  Mux : Mux  Inputs=3
  Product3 : Product
  Solar Radiation Moment - X Axis : Product  Inputs=4
  Solar Radiation Moment - Y  Axis : Product  Inputs=4
  Solar Radiation Moment - Z  Axis : Product  Inputs=4
  SpeedOfLight : Constant  Value=3e8
  Trigonometric Function1 : Trigonometry
  Trigonometric Function2 : Trigonometry  Operator=atan
  Trigonometric Function3 : Trigonometry
  Trigonometric Function4 : Trigonometry  Operator=cos
  SolarRadDistTorque : Outport
  wires:
  DeltaY/1 -> Solar Radiation Moment - Y  Axis/4
  [SolarCoeff] -> Solar Radiation Moment - Y  Axis/2
  [sinForY] -> Solar Radiation Moment - Y  Axis/1
  Ay/1 -> Solar Radiation Moment - Y  Axis/3
  DeltaZ/1 -> Solar Radiation Moment - Z  Axis/4
  DeltaX/1 -> Solar Radiation Moment - X Axis/4
  Ax/1 -> Solar Radiation Moment - X Axis/3
  [cosForX] -> Solar Radiation Moment - X Axis/1
  Trigonometric Function1/1 -> [sinForZ]
  Demux/3 -> Trigonometric Function1/1
  Trigonometric Function3/1 -> [sinForY]
  Trigonometric Function4/1 -> [cosForX]
  Divide1/1 -> [SolarCoeff]
  Fs/1 -> Divide1/1
  (1+kworstCase)/1 -> Divide1/2
  Product3/1 -> Trigonometric Function2/1
  Trigonometric Function2/1 -> Trigonometric Function4/1, Trigonometric Function3/1
  [SolarCoeff] -> Solar Radiation Moment - X Axis/2
  Demux/2 -> Product3/2
  SpeedOfLight/1 -> Divide1/3
  Az/1 -> Solar Radiation Moment - Z  Axis/3
  [SolarCoeff] -> Solar Radiation Moment - Z  Axis/2
  [sinForZ] -> Solar Radiation Moment - Z  Axis/1
  SunPositionVector/1 -> Demux/1
  Demux/1 -> Divide/2
  Constant/1 -> Divide/1
  Divide/1 -> Product3/1
  Solar Radiation Moment - X Axis/1 -> Mux/1  "3x1"
  Solar Radiation Moment - Y  Axis/1 -> Mux/2  "3x1"
  Solar Radiation Moment - Z  Axis/1 -> Mux/3  "3x1"
  Mux/1 -> Display/1, SolarRadDistTorque/1

== system Satellite_Attitude_Model/Satellite Kinematic & Dynamic Model/Kinematic Model1/Subsystem2/Subsystem ==
  q1,q2,q3,q4 : Inport
  Demux1 : Demux
  Mux1 : Mux
  q0,q1,q2,q3 : Outport
  wires:
  Demux1/2 -> Mux1/3
  q1,q2,q3,q4/1 -> Demux1/1
  Mux1/1 -> q0,q1,q2,q3/1
  Demux1/4 -> Mux1/1
  Demux1/1 -> Mux1/2
  Demux1/3 -> Mux1/4

== matlab function Satellite_Attitude_Model/Orbit Propagator Model/Cartesian To Kepler Transform1 ==
  data: r_ECI input; semiMajorAxis output; inclination output; eccNorm output; RAAN output; v_ECI input; argOfPerigee output; trueAnomaly output
function [semiMajorAxis,inclination,eccNorm,RAAN, argOfPerigee,trueAnomaly] = CartesianToKepler(r_ECI, v_ECI)

% (Chobotov pg 66)

% INPUTS
% R_eci  : Satellite position in ECI frame [m]
% dR_eci : Satellite velocity in ECI frame [m/sec]

% OUTPUTS
% a      : Semi major axis [m]
% e      : Eccentricity
% inc    : Inclination [rad]
% RAAN   : Right Ascension of the Ascending Node [rad]
% w      : Argument of Perigee [rad]
% TrAn   : True Anomaly [rad]
semiMajorAxis = 0;
inclination = 0;
eccNorm = 0;
RAAN = 0;
argOfPerigee=0;
trueAnomaly=0;

% Earth Gravitational Constant [ in m3/sec2 ]
mu      = 3.98603e14 ; 
Rn      = norm(  r_ECI ) ;
dRn     = norm( v_ECI ) ;

semiMajorAxis = 1 / (2/Rn - (dRn*dRn)/mu) ; % [m]

WW = cross(r_ECI,v_ECI) / norm(cross(r_ECI,v_ECI));

inclination = acos(dot(WW,[0;0;1])); % [rad]

eccentricity = (1/mu)*((dRn*dRn - mu/Rn)*r_ECI - dot(r_ECI,v_ECI)*v_ECI);

eccNorm = norm(eccentricity);

N = cross([0;0;1],WW) / norm(cross([0;0;1],WW));

cRAAN = dot([1;0;0],N);

sRAAN = dot(cross([1;0;0],N),[0;0;1]);

RAAN = atan2(sRAAN,cRAAN); % [rad]

if eccNorm < 1e-4
    eccNorm = 0; 
%     ecc     = [0; 0; 0];
%     cw      = 0 ;
%     sw      = 0 ;
%     cTrAn   = 0 ;
%     sTrAn   = 0 ;

% Whenever e = 0, argument of perigee and true anomaly are not calculated. 
    argOfPerigee       = 0 ;
    trueAnomaly    = 0 ;
else
    cw = dot(N,eccentricity) / eccNorm ;
    sw = dot((cross(N,eccentricity)/eccNorm),WW) ;
    cTrAn = dot(eccentricity,r_ECI)/(eccNorm*norm(r_ECI)) ;
    sTrAn = dot(cross(eccentricity,r_ECI)/(eccNorm*norm(r_ECI)),WW) ;
    argOfPerigee = atan2(sw,cw); % [rad]
    trueAnomaly = atan2(sTrAn, cTrAn) ; % [rad]
end

== matlab function Satellite_Attitude_Model/Orbit Propagator Model/MATLAB Function ==
  data: r_ECI input; r_ECEF output; times input
%% function 'eci2ecef_multitime'
%
% Transforms coordinates in ECI to coordinates in ECEF
% ECI : Earth Centered Inertial Frame
% ECEF: Earth Centered Earth Fixed Frame
%
% Input  : pos_eci  = [x; y; z] | ECI                      [m]
%          times    = times since vernal equinox alignment [s]
% Output : pos_ecef = [x; y; z] | ECEF                     [m]

function r_ECEF = eci2ecef(r_ECI, times)

% This is the rotation rate of Earth (rad/s)
w_earth = 7.292115e-5;

% Initialise varibles
angles = w_earth*times;
c      = cos(angles);
s      = sin(angles);

% % Tranformation Matrix
% eci2ecefTranform = [c s 0; -s c 0; 0 0 1];
% 
% % Final Transformation 
% pos_ecef = eci2ecefTranform * pos_eci;

% Find ECI Coordinates
r_ECEF = zeros(3,1);
r_ECEF(1,:) =  r_ECI(1,:).*c + r_ECI(2,:).*s; 
r_ECEF(2,:) = -r_ECI(1,:).*s + r_ECI(2,:).*c;
r_ECEF(3,:) =  r_ECI(3,:);

end

== matlab function Satellite_Attitude_Model/Orbit Propagator Model/MATLAB Function1 ==
  data: r_ECEF input; lat_rad output; lon_rad output; h_m output
function [lat_rad, lon_rad, h_m] = ecef2LLA(r_ECEF)
% Input  : [x; y; z]         [m]
% Output : [lat;long;alt]    [rad,rad,m]
%--------------------------------------------------------------------------

r_earth = 6378137;
   
% Initialise ECEF Coordinates
x = r_ECEF(1,:);
y = r_ECEF(2,:);
z = r_ECEF(3,:);

% Finding vector magnitutde
R  =  sqrt(x.^2 + y.^2 + z.^2);

% Calculate geocentric lattitude
lat_rad = asin(z./R);

% Calculate geocentric longitude 
lon_rad     = atan2(y,x);

% Calculate altitude 
h_m = R - r_earth;

% Return geocentric coordinates
% LLA = [lat_c;long;alt];

end


% function [lat_deg, lon_deg, h_km] = ECEF2LLA(rEcef)
% %--------------------------------------------------------------------------
% %   From Earth fixed cartesian to latitude, longitude and altitude
% %--------------------------------------------------------------------------
% %   Form:
% %   [lat, lon, h] = ECEF2LLH(rEcef)
% %--------------------------------------------------------------------------
% %   Inputs
% %   rEcef           (3,1)   ECEF position
% %--------------------------------------------------------------------------
% %   Outputs
% %   lat             (1,1)   Latitude(deg)
% %   lon             (1,1)   Longitude(deg)
% %   h               (1,1)   Altitude(km)
% %--------------------------------------------------------------------------
% 
% a    = 6378137.0;
% finv = 298.257223563;
% f    = 1/finv;
% e2   = 1-(1-f)^2;
% 
% X = rEcef(1)*1000;
% Y = rEcef(2)*1000;
% Z = rEcef(3)*1000;
% 
% % Latitude and height convergence criteria
% elat=1.e-3;
% eht=1.e-3;
% 
% % Initial values for iteration
% p=sqrt(X.*X+Y.*Y);
% lat=atan2(Z,p.*(1-e2));
% h=0;
% dh=1;
% dlat=1;
% 
% % Iterate until lat & h converge to elat & eht
% while sum(dlat>elat) || sum(dh>eht)
%     lat0=lat;
%     h0=h;
%     v=a./sqrt(1-e2.*sin(lat).*sin(lat));
%     h=p./cos(lat)-v;
%     lat=atan2(Z, p.*(1-e2.*v./(v+h)));
%     dlat=abs(lat-lat0);
%     dh=abs(h-h0);
% end
% lon=atan2(Y,X);
% lon_deg = lon*180/pi;
% lat_deg = lat*180/pi;
% h_km = h/1000;

== matlab function Satellite_Attitude_Model/Satellite Kinematic & Dynamic Model/Dynamic Model/Embedded MATLAB Function ==
  data: w input; y output; Iw_plus_hwheel input
function y = crossproduct(w,Iw_plus_hwheel)
% This block supports the Embedded MATLAB subset.
% See the help menu for details. 

%Just used to calculate the cross-product of two inputs
y = cross(w,Iw_plus_hwheel);

== matlab function Satellite_Attitude_Model/Julian Date Model/Time To Julian Date Model/Date To Julian Date Model ==
  data: time input; JD output
function JD = dt2jd( time )
% INPUTS
% Calendar Date : The date & time to be converted to JD in
%                 [ year ; month ; day ; hour ; minute ; second ]
%                 format.
%
% OUTPUTS
% JD            : Julian Date as defined in "Spacecraft Mission Design,
%                 by Charles Brown, 2nd edition, AIAA", pp. 31
% T             : Number of Julian Centuries

year    = time(1) ;
month   = time(2) ;
day     = time(3) ;
hour    = time(4) ;
minute  = time(5) ;
second  = time(6) ;

% Day fraction due to given time
day_fr  = (hour*3600 + minute*60 + second)/86400 ;

day     = day + day_fr;

% Julian Date
JD      = 367*year-floor(7*(year+floor((month+9)/12))/4) +...
                   floor((275*month)/9)+day+1721013.5 ;

== matlab function Satellite_Attitude_Model/Orbit Propagator Model/MATLAB Function2 ==
  data: h input; w_IO_O output
function w_IO_O = fcn(h)


mu = 398600.4418e9; % m^3/s^2
Re = 6378000; % m
w_IO_O = sqrt(mu/(Re+h)^3); % 1/s

% w_IO_O = w_IO_O * 2*pi/86400;

end

== matlab function Satellite_Attitude_Model/Satellite Kinematic & Dynamic Model/Kinematic Model1/Subsystem2/MATLAB Function ==
  data: DCM input; DCM_2 output
function DCM_2 = fcn(DCM)
DCM_2 = DCM(:,2);
end

== matlab function Satellite_Attitude_Model/Orbit Propagator Model/Orbit Propagator Model with Kepler Parameters(ECI)/J2 Propagator Model ==
  data: semimajor input; inclination input; RAAN_dot output; eccentricity input; ArgOfPerigee_dot output; meanMotion output; n input
function [ RAAN_dot, ArgOfPerigee_dot, meanMotion ] = J2propagator (semimajor, inclination, eccentricity, n)

% Orbit Propagator with J2 perturbation 
% Chobotov - Orbital Mechanics Third Edition
%--------------------------------------------------------------
% INPUTS
%--------------------------------------------------------------
% semimajor     = semimajor axis [m]
% eccentricity  = eccentricity
% inclination   = inclination [rad]
%--------------------------------------------------------------
% OUTPUTS
%--------------------------------------------------------------
% raand = time derivative of RAAN [rad/s]
% omgd  = time derivative of Argument of Perigee [rad/s]
% Md = time derivative of Mean Anomaly [rad/s]

%  mu = GM for the Earth (m^3/s^2)
% mu_earth = 398600.4418e9;
% The J2 correction constant
J2 = 0.00108262668;
% The radius of the Earth (m)
r_earth = 6378137;

% earth_mu    = 3.98603e14;  % Earth Gravitational Constant [ in m3/sec2 ]
% Re          = 6.378137e6 ; % earth equatorial radius [in meters ]
% J2          = 1.08263e-3;  % the second gravitational zonal harmonic of Earth

% Semilatus Rectum [m]
p = semimajor*(1- eccentricity^2); 

% mean motion [1/s]
% n = sqrt(mu_earth/semimajor^3); 

% Orbit Mean Motion with J2 correction [1/s]
nt = n + 1.5 * n * J2 * (r_earth/p)^2 * ( 1 - 1.5 * sin(inclination)^2) *sqrt(1-eccentricity^2);

% Time Derivatiove of  RAAN [rad/s]
RAAN_dot = -1.5 * nt * J2 * (r_earth/p)^2 * cos(inclination);

% Time Derivatiove of Argument of Perigee [rad/s]
ArgOfPerigee_dot = 0.75*nt*J2*(r_earth/p)^2*(2-2.5*sin(inclination)^2);

% Time Derivative of Mean Anomaly [rad/s]
% MeanAnomaly_dot = nt;
meanMotion = nt;
% meanMotion = meanMotion*2*pi/86400; % rad/sn
